simulink model "PKE_NoFeedback"  (R2020a)
settings: Solver=ode15s  StartTime=0.0  StopTime=300  RelTol=1e-5
model workspace (MAT data in the model file):
  B = [1 1 1 1 1 1]
  Be = 1
  Co = [1 1 1 1 1 1]
  Gt = 1
  PoMW = 0
  lam = [1 1 1 1 1 1]
  rho = 1
undefined symbols (not defined in the file): Po
settings Model: OrderedModelArguments=off  Creator=Joel_Strandburg  LastModifiedBy=jts53
settings SFSimCC: CustomCodeUndefinedFunction=UseInterfaceOnly

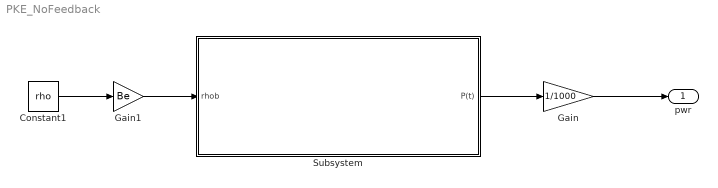
== system PKE_NoFeedback ==
  Constant1 : Constant  Value=rho
  Gain : Gain  Gain=1/1000
  Gain1 : Gain  Gain=Be
  Subsystem : Subsystem
  pwr : Outport
  wires:
  Subsystem/1(P(t)) -> Gain/1
  Constant1/1 -> Gain1/1
  Gain1/1 -> Subsystem/1(rhob)
  Gain/1 -> pwr/1

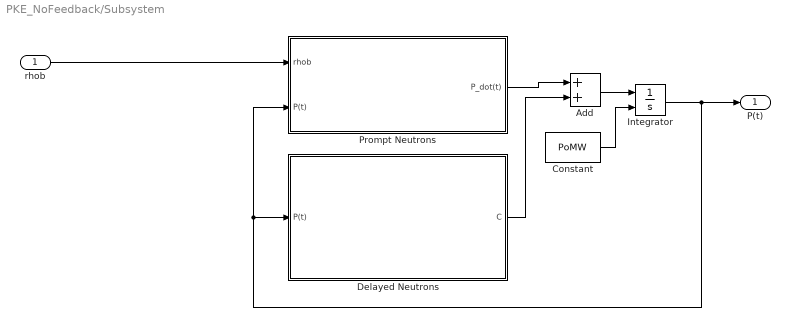
== system PKE_NoFeedback/Subsystem ==
  rhob : Inport
  Add : Sum
  Constant : Constant  Value=PoMW
  Delayed Neutrons : Subsystem
  Integrator : Integrator  InitialConditionSource=external  InitialCondition=PoMW*1e6
  Prompt Neutrons : Subsystem
  P(t) : Outport  VectorParamsAs1DForOutWhenUnconnected=off
  wires:
  Add/1 -> Integrator/1
  rhob/1 -> Prompt Neutrons/1(rhob)
  Integrator/1 -> P(t)/1, Prompt Neutrons/2(P(t)), Delayed Neutrons/1(P(t))
  Constant/1 -> Integrator/2
  Delayed Neutrons/1(C) -> Add/2
  Prompt Neutrons/1(P_dot(t)) -> Add/1

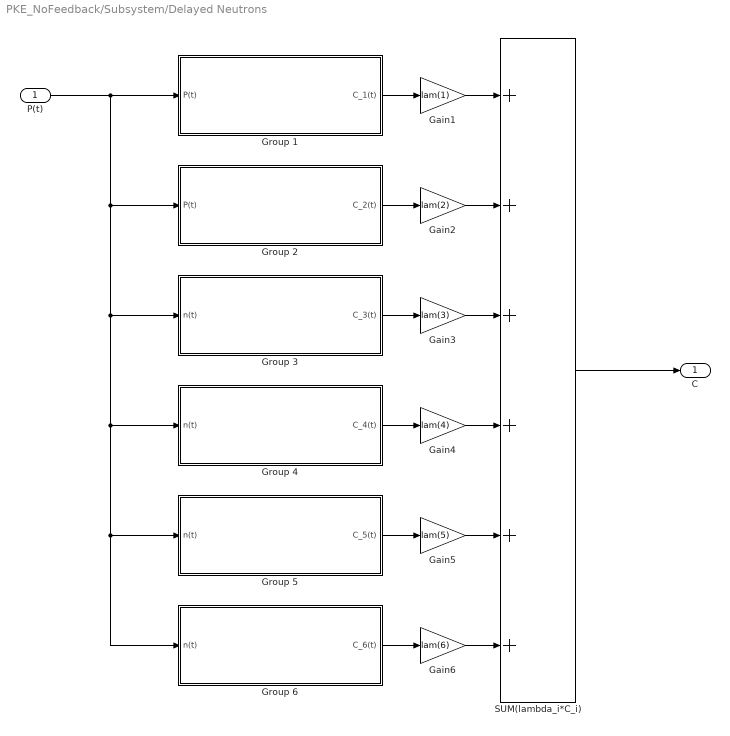
== system PKE_NoFeedback/Subsystem/Delayed Neutrons ==
  P(t) : Inport
  Gain1 : Gain  Gain=lam(1)
  Gain2 : Gain  Gain=lam(2)
  Gain3 : Gain  Gain=lam(3)
  Gain4 : Gain  Gain=lam(4)
  Gain5 : Gain  Gain=lam(5)
  Gain6 : Gain  Gain=lam(6)
  Group 1 : Subsystem
  Group 2 : Subsystem
  Group 3 : Subsystem
  Group 4 : Subsystem
  Group 5 : Subsystem
  Group 6 : Subsystem
  SUM(lambda_i*C_i) : Sum  Inputs=++++++
  C : Outport  VectorParamsAs1DForOutWhenUnconnected=off
  wires:
  P(t)/1 -> Group 6/1(n(t)), Group 5/1(n(t)), Group 4/1(n(t)), Group 3/1(n(t)), Group 2/1(P(t)), Group 1/1(P(t))
  SUM(lambda_i*C_i)/1 -> C/1
  Group 1/1(C_1(t)) -> Gain1/1
  Gain1/1 -> SUM(lambda_i*C_i)/1
  Gain2/1 -> SUM(lambda_i*C_i)/2
  Group 2/1(C_2(t)) -> Gain2/1
  Group 3/1(C_3(t)) -> Gain3/1
  Gain3/1 -> SUM(lambda_i*C_i)/3
  Group 4/1(C_4(t)) -> Gain4/1
  Gain4/1 -> SUM(lambda_i*C_i)/4
  Group 5/1(C_5(t)) -> Gain5/1
  Gain5/1 -> SUM(lambda_i*C_i)/5
  Group 6/1(C_6(t)) -> Gain6/1
  Gain6/1 -> SUM(lambda_i*C_i)/6

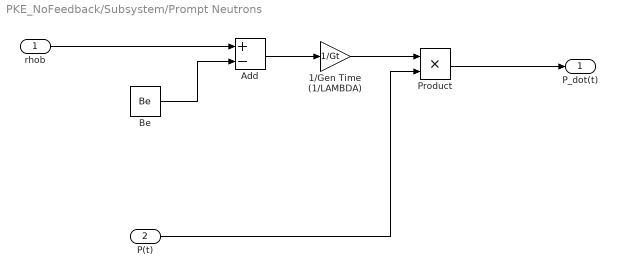
== system PKE_NoFeedback/Subsystem/Prompt Neutrons ==
  rhob : Inport
  P(t) : Inport  Port=2
  1/Gen Time (1/LAMBDA) : Gain  Gain=1/Gt
  Add : Sum  Inputs=+-
  Be : Constant  Value=Be
  Product : Product
  P_dot(t) : Outport  VectorParamsAs1DForOutWhenUnconnected=off
  wires:
  rhob/1 -> Add/1
  Be/1 -> Add/2
  Add/1 -> 1/Gen Time (1/LAMBDA)/1
  1/Gen Time (1/LAMBDA)/1 -> Product/1
  Product/1 -> P_dot(t)/1
  P(t)/1 -> Product/2

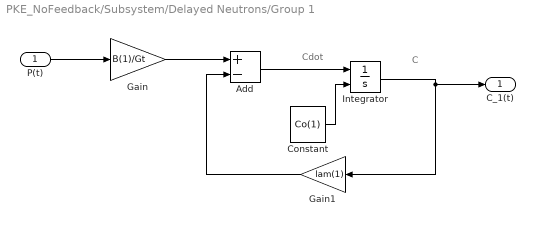
== system PKE_NoFeedback/Subsystem/Delayed Neutrons/Group 1 ==
  note: Cdot
  note: C
  P(t) : Inport
  Add : Sum  Inputs=+-
  Constant : Constant  Value=Co(1)
  Gain : Gain  Gain=B(1)/Gt
  Gain1 : Gain  Gain=lam(1)
  Integrator : Integrator  InitialConditionSource=external  InitialCondition=B(1)*Po./(lam(1)*Gt)
  C_1(t) : Outport  VectorParamsAs1DForOutWhenUnconnected=off
  wires:
  P(t)/1 -> Gain/1
  Gain/1 -> Add/1
  Add/1 -> Integrator/1
  Integrator/1 -> Gain1/1, C_1(t)/1
  Gain1/1 -> Add/2
  Constant/1 -> Integrator/2

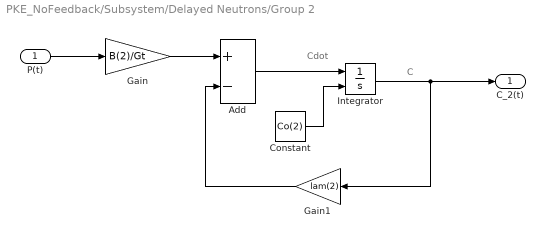
== system PKE_NoFeedback/Subsystem/Delayed Neutrons/Group 2 ==
  note: Cdot
  note: C
  P(t) : Inport
  Add : Sum  Inputs=+-
  Constant : Constant  Value=Co(2)
  Gain : Gain  Gain=B(2)/Gt
  Gain1 : Gain  Gain=lam(2)
  Integrator : Integrator  InitialConditionSource=external  InitialCondition=B(2)*Po./(lam(2)*Gt)
  C_2(t) : Outport  VectorParamsAs1DForOutWhenUnconnected=off
  wires:
  P(t)/1 -> Gain/1
  Add/1 -> Integrator/1
  Integrator/1 -> Gain1/1, C_2(t)/1
  Constant/1 -> Integrator/2
  Gain1/1 -> Add/2
  Gain/1 -> Add/1

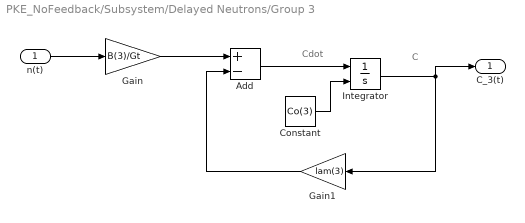
== system PKE_NoFeedback/Subsystem/Delayed Neutrons/Group 3 ==
  note: Cdot
  note: C
  n(t) : Inport
  Add : Sum  Inputs=+-
  Constant : Constant  Value=Co(3)
  Gain : Gain  Gain=B(3)/Gt
  Gain1 : Gain  Gain=lam(3)
  Integrator : Integrator  InitialConditionSource=external  InitialCondition=B(3)*Po./(lam(3)*Gt)
  C_3(t) : Outport  VectorParamsAs1DForOutWhenUnconnected=off
  wires:
  n(t)/1 -> Gain/1
  Gain/1 -> Add/1
  Add/1 -> Integrator/1
  Integrator/1 -> C_3(t)/1, Gain1/1
  Gain1/1 -> Add/2
  Constant/1 -> Integrator/2

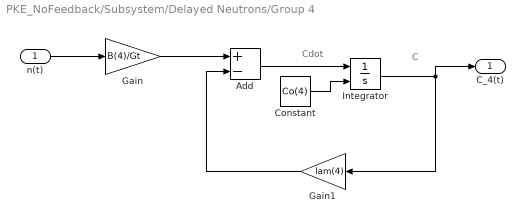
== system PKE_NoFeedback/Subsystem/Delayed Neutrons/Group 4 ==
  note: Cdot
  note: C
  n(t) : Inport
  Add : Sum  Inputs=+-
  Constant : Constant  Value=Co(4)
  Gain : Gain  Gain=B(4)/Gt
  Gain1 : Gain  Gain=lam(4)
  Integrator : Integrator  InitialConditionSource=external  InitialCondition=B(4)*Po./(lam(4)*Gt)
  C_4(t) : Outport  VectorParamsAs1DForOutWhenUnconnected=off
  wires:
  n(t)/1 -> Gain/1
  Gain/1 -> Add/1
  Add/1 -> Integrator/1
  Integrator/1 -> C_4(t)/1, Gain1/1
  Gain1/1 -> Add/2
  Constant/1 -> Integrator/2

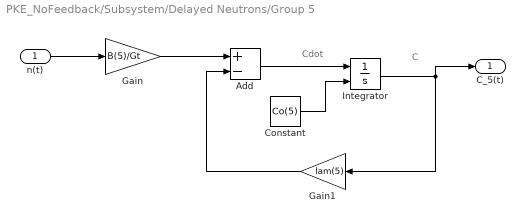
== system PKE_NoFeedback/Subsystem/Delayed Neutrons/Group 5 ==
  note: Cdot
  note: C
  n(t) : Inport
  Add : Sum  Inputs=+-
  Constant : Constant  Value=Co(5)
  Gain : Gain  Gain=B(5)/Gt
  Gain1 : Gain  Gain=lam(5)
  Integrator : Integrator  InitialConditionSource=external  InitialCondition=B(5)*Po./(lam(5)*Gt)
  C_5(t) : Outport  VectorParamsAs1DForOutWhenUnconnected=off
  wires:
  n(t)/1 -> Gain/1
  Gain/1 -> Add/1
  Add/1 -> Integrator/1
  Integrator/1 -> C_5(t)/1, Gain1/1
  Gain1/1 -> Add/2
  Constant/1 -> Integrator/2

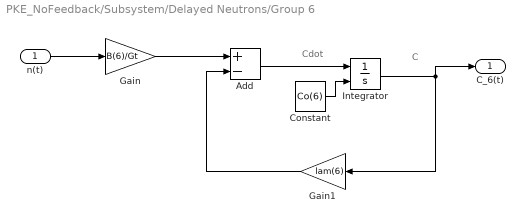
== system PKE_NoFeedback/Subsystem/Delayed Neutrons/Group 6 ==
  note: Cdot
  note: C
  n(t) : Inport
  Add : Sum  Inputs=+-
  Constant : Constant  Value=Co(6)
  Gain : Gain  Gain=B(6)/Gt
  Gain1 : Gain  Gain=lam(6)
  Integrator : Integrator  InitialConditionSource=external  InitialCondition=B(6)*Po./(lam(6)*Gt)
  C_6(t) : Outport  VectorParamsAs1DForOutWhenUnconnected=off
  wires:
  n(t)/1 -> Gain/1
  Gain/1 -> Add/1
  Add/1 -> Integrator/1
  Integrator/1 -> C_6(t)/1, Gain1/1
  Gain1/1 -> Add/2
  Constant/1 -> Integrator/2
